simulink model "Ex_04_PD_Control_Plus_Feedforward"  (Simulink 8.9)
settings: Solver=ode3  StartTime=0.0  StopTime=t_max  FixedStep=jointObj.Ts  RelTol=1e-3  EnableMultiTasking=on
values from neighbouring files (symbols this model uses):
  t_max = f_max    (= 100)    [Ex_00_example_config.m]
libraries: simulink x1, cjt_library_models x1, cjt_library_controllers x1
settings Model: SuppressorTable=22 serialization::archive 11 0 6 0 0 0 11 0  Creator=joern  LastModifiedBy=wesley
settings DataIOCC: LimitDataPoints=off  SignalLoggingSaveFormat=Dataset
settings DebuggingCC: UnderspecifiedInitializationDetection=Simplified  MergeDetectMultiDrivingBlocksExec=error  SolverPrmCheckMsg=warning  FcnCallInpInsideContextMsg=error  StateNameClashWarn=none
settings GRTTargetCC: CombineOutputUpdateFcns=on  GRTInterface=off
settings ConfigComp: CovSFcnEnable=off

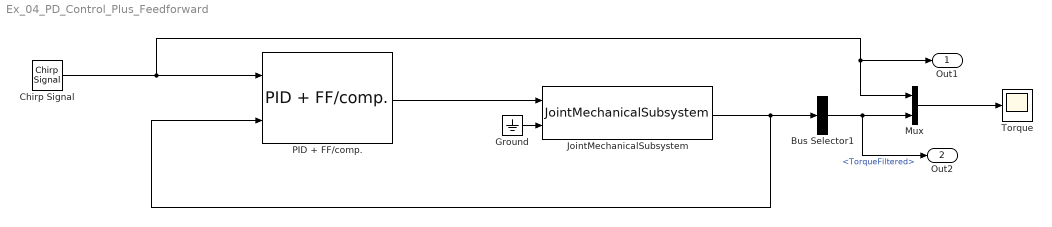
== system Ex_04_PD_Control_Plus_Feedforward ==
  Bus Selector1 : BusSelector  OutputSignals=TorqueFiltered
  Chirp Signal : simulink/Sources/Chirp Signal  f1=f_min  T=t_max  f2=f_max
  Ground : Ground
  JointMechanicalSubsystem : cjt_library_models/Joint models/JointMechanicalSubsystem  jointObj=jointObj  fc_vel=499  fc_torque=499  input_delay=1  output_delay=1  quantize=on  quantize_bits=19  input_noise_enabled=off  output_noise_enabled=off  var_u=0.12^2  var_y=1.8e-10
  Mux : Mux  Inputs=2
  PID + FF/comp. : cjt_library_controllers/Controllers/PID + FF//comp.  jointObj=jointObj  Kp=0  Ki=0  Kd=0  N=2*pi*200  ff_comp_switch=Feed-forward
  Torque : Scope
  Out1 : Outport
  Out2 : Outport  Port=2
  wires:
  Mux/1 -> Torque/1
  Ground/1 -> JointMechanicalSubsystem/2
  JointMechanicalSubsystem/1 -> PID + FF/comp./2, Bus Selector1/1
  PID + FF/comp./1 -> JointMechanicalSubsystem/1
  Chirp Signal/1 -> PID + FF/comp./1, Out1/1, Mux/1
  Bus Selector1/1 -> Out2/1, Mux/2  "<TorqueFiltered>"

== matlab function JointMechanicalSubsystem/nonLinDynamicsFcn ==
  data: x input double; tau output double
function tau = nonLinDynamics(x)
%#codegen

params.a_CU = 0.003900;
params.c_CU = 380.000000;
params.c_FE = 460.000000;
params.diam = 93.000000;
params.len = 163.000000;
params.m = 1.450000;
params.I_m = 0.229997;
params.I_g = 0.071680;
params.I_l = 0.000114;
params.k_g = 16000.000000;
params.k_b = 6000.000000;
params.d_m = 0.003592;
params.d_g = 0.384000;
params.d_l = 0.000000;
params.d_m_n = 0.003592;
params.d_g_n = 0.384000;
params.d_l_n = 0.000000;
params.d_mg = 100.000000;
params.d_gl = 0.000000;
params.d_cm = 2.640000;
params.d_cg = 3.280000;
params.d_cl = 0.000000;
params.d_cm_n = 2.640000;
params.d_cg_n = 3.280000;
params.d_cl_n = 0.000000;
params.d_s = 0.000000;
params.v_s = 0.000000;
params.rip_types = [];
params.rip_a1 = [];
params.rip_a2 = [];
params.rip_f = [];
params.n = 80.000000;
params.k_t = 0.078000;
params.r = 0.318000;
params.x = 0.000200;
params.v_0 = 48.000000;
params.i_p = 33.900000;
params.dq_p = 7.728395;
params.r_th1 = 3.136441;
params.r_th2 = 32.663680;
params.T_thw = 98.081750;
params.T_thm = 4679.965000;
params.Tmp_WMax = 155.000000;
params.Tmp_ANom = 25.000000;
params.name = 'example_joint_locked';
params.paramName = 'cjt_Orange_80_6000';
params.modelName = 'output_fixed';
params.nonlinearModelName = 'coulomb_asym';
params.Ts = 0.001000;
params.Ts_elec = 0.000050;
tau =coulomb_asym(params,x);
	end
